simulink model "ThreePhaseASMSaturation"  (R2023b)
settings: Solver=ode23tb  StartTime=0.0  StopTime=3.5  MaxStep=1/60  RelTol=1e-4  AbsTol=1e-4  EnableMultiTasking=on
InitFcn:
  | run('DefaultSimscapeValues.m')
values from neighbouring files (symbols this model uses):
  D = 0    [DefaultSimscapeValues.m]    (also in Newabccoordparam.m = 0.001)
  f = 60    [DefaultSimscapeValues.m]    (also in Newabccoordparam.m = 50)
  J = 1.662    [DefaultSimscapeValues.m]    (also in Newabccoordparam.m = 127)
  Lm = 13.08/377    (= 0.0346949602122)    [DefaultSimscapeValues.m]    (also in Newabccoordparam.m = 0.0025)
  Lr = Lm + Lsi    (= 0.0354960212202)    [DefaultSimscapeValues.m]    (also in Newabccoordparam.m = 0.002587)
  Lri = 0.302/377    (= 0.000801061007958)    [DefaultSimscapeValues.m]    (also in Newabccoordparam.m = 8.7e-05)
  Ls = Lm + Lsi    (= 0.0354960212202)    [DefaultSimscapeValues.m]    (also in Newabccoordparam.m = 0.002587)
  Lsi = 0.302/377    (= 0.000801061007958)    [DefaultSimscapeValues.m]    (also in Newabccoordparam.m = 8.7e-05)
  p = 2    [DefaultSimscapeValues.m]    (also in Newabccoordparam.m)
  Ps = 37300    [DefaultSimscapeValues.m]    (also in Newabccoordparam.m = 2000000)
  Rr = 0.228    [DefaultSimscapeValues.m]    (also in Newabccoordparam.m = 0.0029)
  Rs = 0.087    [DefaultSimscapeValues.m]    (also in Newabccoordparam.m = 0.0026)
  sigma = 1- Lm^2/(Ls*Lr)    (= 0.0446259584738)    [DefaultSimscapeValues.m]    (also in Newabccoordparam.m = 0.0661284179513)
  Vs = 460    [DefaultSimscapeValues.m]    (also in Newabccoordparam.m = 690)
undefined symbols (not defined in the file or in its folder): DiscIntNeverNeededParam
libraries: eeGeneralControl x4, spsabctodq0Lib x4, spsdq0toabcLib x4, spsAsynchronousMachineSIUnitsLib x2, spsThreePhaseProgrammableVoltageSourceLib x1, spsGroundLib x1, sps_lib x1
settings Model: FPTRunName=Active  Creator=The MathWorks, Inc.  LastModifiedBy=collins
settings SolverCC: AutoScaleAbsTol=off  AlgebraicLoopSolver=TrustRegion
settings DataIOCC: LimitDataPoints=on  SaveFormat=Array  ReturnWorkspaceOutputs=off
settings OptimizationCC: ExpressionDepthLimit=2147483647  InitFltsAndDblsToZero=on  EfficientMapNaN2IntZero=off  LifeSpan=inf
settings DebuggingCC: UnderspecifiedInitializationDetection=Classic  MergeDetectMultiDrivingBlocksExec=none  SignalResolutionControl=TryResolveAllWithWarning  SolverPrmCheckMsg=warning  MultiTaskDSMMsg=warning  MultiTaskCondExecSysMsg=none  SigSpecEnsureSampleTimeMsg=none  FcnCallInpInsideContextMsg=warning  UnconnectedInputMsg=warning  UnconnectedOutputMsg=warning  UnconnectedLineMsg=warning  StateNameClashWarn=warning  SFUnexpectedBacktrackingDiag=warning  SFNoUnconditionalDefaultTransitionDiag=warning  SFExecutionAtInitializationDiag=none  ArithmeticOperatorsInVariantConditions=warning
settings HardwareCC: ProdBitPerPointer=32  ProdBitPerSizeT=32  ProdBitPerPtrDiffT=32  ProdLargestAtomicFloat=None  ProdIntDivRoundTo=Undefined  ProdEndianess=Unspecified  ProdWordSize=32  ProdHWDeviceType=32-bit Generic
settings ModelReferenceCC: EnableRefExpFcnMdlSchedulingChecks=on  PropagateSignalLabelsOutOfModel=off
settings SFSimCC: SimUseLocalCustomCode=off  CustomCodeUndefinedFunction=UseInterfaceOnly
settings RTWCC: RTWUseLocalCustomCode=off  DLArmComputeVersion=19.05
settings CodeAppCC: StateflowObjectComments=on
settings GRTTargetCC: TargetLangStandard=C89/C90 (ANSI)  CombineOutputUpdateFcns=off  GRTInterface=on
settings ConfigComp: CovMetricSettings=dw  CovSaveCumulativeToWorkspaceVar=on  CovSaveSingleToWorkspaceVar=on  CovExternalEMLEnable=off  CovSFcnEnable=off
settings SimscapeCC: SimscapeNormalizeSystem=off

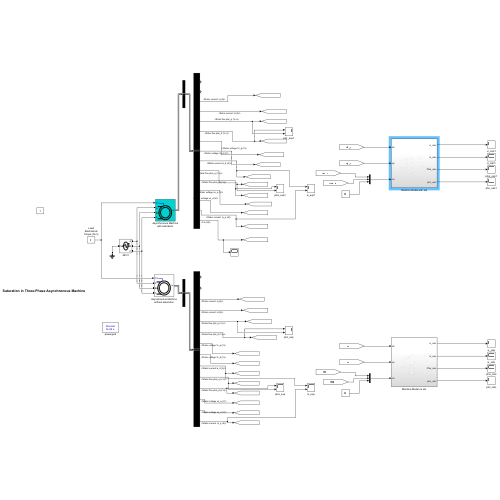
[thumbnail: Simulink's stored preview of the top-level diagram]
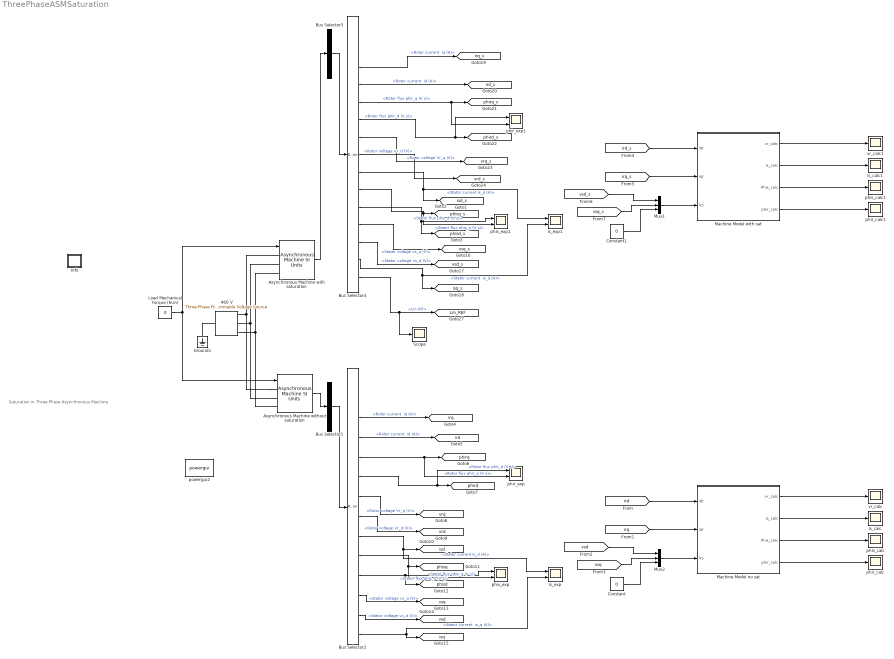
== system ThreePhaseASMSaturation ==
  note: Saturation in Three-Phase Asynchronous Machine
  460 V : spsThreePhaseProgrammableVoltageSourceLib/Three-Phase Programmable Voltage Source  PositiveSequence="[460  0 60]"  VariationEntity=None  VariationType=Step  VariationTypeAlt=Step  VariationStep=0.5  VariationRate=10  VariationMagnitude=0.3  VariationFrequency=2  VariationTiming=[1 2]  VariationPhaseA=off  Amplitudes=[1 0.8 1.2 1.0]  TimeValues=[0 0.1 0.15 0.2]  HarmonicGeneration=off  HarmonicA=[3 0.2 -25 0]  HarmonicB=[2 0.15 35 2]  Timing="[0.05  3]"  BusType=swing  Pref=0  Qref=0  Qmin=-inf  Qmax=inf
  Asynchronous Machine with saturation : spsAsynchronousMachineSIUnitsLib/Asynchronous Machine SI Units  RotorType=Squirrel-cage  PresetModel=No  MechanicalLoad=Torque Tm  ShowDetailedParameters=on  ReferenceFrame=Synchronous  Units=SI  MeasurementBus=off  NominalParameters=[Ps Vs f]  VoltageRatio=1  Stator=[Rs Lsi]  Rotor=[Rr Lri]  Cage1=[ 0.022 0.226/377]  Cage2=[ 0.022 0.226/377]  Lm=13.08/377  Mechanical=[J D p]  PolePairs=2  InitialConditions="[ 1,0   0,0,0   0,0,0 ]"  SimulateSaturation=on  Saturation=[9.9249,19.6672,38.0377,51.3988,69.2824,105.1337,152.5532,214.2421,302;230, 322, 414, 460, 506, 552, 598, 644, 690]  LoadFlowParameters=0  TsPowergui=0  TsBlock=-1  IterativeModel=Trapezoidal non iterative  IterativeDiscreteModel=Trapezoidal non iterative  Pmec=0
  Asynchronous Machine without saturation : spsAsynchronousMachineSIUnitsLib/Asynchronous Machine SI Units  RotorType=Squirrel-cage  PresetModel=No  MechanicalLoad=Torque Tm  ShowDetailedParameters=on  ReferenceFrame=Synchronous  Units=SI  MeasurementBus=off  NominalParameters=[Ps Vs f]  VoltageRatio=1  Stator=[Rs Lsi]  Rotor=[Rr Lri]  Cage1=[ 0.022 0.226/377]  Cage2=[ 0.022 0.226/377]  Lm=Lm  Mechanical=[J D p]  PolePairs=2  InitialConditions=[ 1,0,0,0,0,0,0,0 ]  SimulateSaturation=off  Saturation=[9.9249,19.6672,38.0377,51.3988,69.2824,105.1337,152.5532,214.2421,302;230, 322, 414, 460, 506, 552, 598, 644, 690]  LoadFlowParameters=0  TsPowergui=0  TsBlock=-1  IterativeModel=Trapezoidal non iterative  IterativeDiscreteModel=Trapezoidal non iterative  Pmec=0
  Bus Selector1 : BusSelector  OutputSignals="Stator measurements.Stator current is_a (A),Mechanical.Rotor speed (wm),Rotor measurements.Rotor current  iq (A),Rotor measurements.Rotor current  id (A),Rotor measurements.Rotor flux phir_q (V s),Rotor measurements.Rotor flux phir_d (V s),Rotor measurements.Rotor voltage Vr_q (V),Rotor measurements.Rotor voltage Vr_d (V),Stator measurements.Stator current is_d (A),Stator measurements.Stator flux phis_q (V s),Stator measurements.Stator flux phis_d (V s),Stator measurements.Stator voltage vs_q (V),Stator measurements.Stator voltage vs_d (V),Stator measurements.Stator current  is_q (A)"  OutputAsBus=on
  Bus Selector2 : BusSelector  OutputSignals="Stator current is_a (A),Rotor speed (wm),Rotor current  iq (A),Rotor current  id (A),Rotor flux phir_q (V s),Rotor flux phir_d (V s),Rotor voltage Vr_q (V),Rotor voltage Vr_d (V),Stator current is_d (A),Stator flux phis_q (V s),Stator flux phis_d (V s),Stator voltage vs_q (V),Stator voltage vs_d (V),Stator current  is_q (A)"
  Bus Selector3 : BusSelector  OutputSignals="Stator measurements.Stator current is_a (A),Mechanical.Rotor speed (wm),Rotor measurements.Rotor current  iq (A),Rotor measurements.Rotor current  id (A),Rotor measurements.Rotor flux phir_q (V s),Rotor measurements.Rotor flux phir_d (V s),Rotor measurements.Rotor voltage Vr_q (V),Rotor measurements.Rotor voltage Vr_d (V),Stator measurements.Stator current is_d (A),Stator measurements.Stator flux phis_q (V s),Stator measurements.Stator flux phis_d (V s),Stator measurements.Stator voltage vs_q (V),Stator measurements.Stator voltage vs_d (V),Stator measurements.Stator current  is_q (A),Lm (H)"  OutputAsBus=on
  Bus Selector4 : BusSelector  OutputSignals="Stator current is_a (A),Rotor speed (wm),Rotor current  iq (A),Rotor current  id (A),Rotor flux phir_q (V s),Rotor flux phir_d (V s),Rotor voltage Vr_q (V),Rotor voltage Vr_d (V),Stator current is_d (A),Stator flux phis_q (V s),Stator flux phis_d (V s),Stator voltage vs_q (V),Stator voltage vs_d (V),Stator current  is_q (A),Lm (H)"
  Constant : Constant  Value=0
  Constant1 : Constant  Value=0
  Ground1 : spsGroundLib/Ground  LConnTagsString=a
  Info : Subsystem
      settings: OpenFcn="showExample(\"simscapeelectricalsps/ThreePhaseASMSaturationExample\")"
      mask Display: disp('?')
  Load Mechanical Torque (N.m) : Constant  Value=0
  Machine Model no sat : Subsystem
  Machine Model with sat : Subsystem
  Mux1 : Mux  Inputs=3
  Mux2 : Mux  Inputs=3
  Scope : Scope
  is_calc : Scope
  is_calc1 : Scope
  is_exp : Scope  NumInputPorts=2
  is_exp1 : Scope  NumInputPorts=2
  phir_calc : Scope
  phir_calc1 : Scope
  phir_exp : Scope  NumInputPorts=2
  phir_exp1 : Scope  NumInputPorts=2
  phis_calc : Scope
  phis_calc1 : Scope
  phis_exp : Scope  NumInputPorts=2
  phis_exp1 : Scope  NumInputPorts=2
  powergui2 : sps_lib/powergui  Priority=1  SimulationMode=Discrete  SampleTime=5e-6  frequency=60  Iterations=50  frequencyindice=60  Pbase=100e6  ErrMax=1e-4  UnitsV=kV  UnitsW=MW  buscounter=0  FunctionMessages=off  echomessages=off  EnableUseOfTLC=off  CurrentSourceSwitches=off  DisableSnubberDevices=off  DisableRonSwitches=off  DisableVfSwitches=off  DisplayEquations=off  AutomaticDiscreteSolvers=off  SolverType=Tustin  Interpol=off  ExternalGateDelay=off  methode=off  Ts=0  x0status=blocks  SPID=off  SwTol=0  HookPort=off  NonlinearTolerance=1e-4  nMaxIteration=100  ContinueOnMaxIteration=off  RestoreLinks=warning  ResistiveCurrentMeasurement=off  Frange=[0:2:500]  Ylog=off  Xlog=on  ShowGrid=off  save=off  variable=ZData  structure=0  ZoomFFT=off  StartTime=0.0  cycles=1  DisplayStyle=1  fundamental=60  FreqAxis=off  MaxFrequency=1000  frequencyindicesteady=1  RmsSteady=1  display=off
  vr_calc : Scope
  vr_calc1 : Scope
  tag scope: Lm_REF=global, ird=global, ird_s=global, irq=global, irq_s=global, isd=global, isd_s=global, isq=global, isq_s=global, phird=global, phird_s=global, phirq=global, phirq_s=global, phisd=global, phisd_s=global, phisq=global, phisq_s=global, vrd=global, vrd_s=global, vrq=global, vrq_s=global, vsd=global, vsd_s=global, vsq=global, vsq_s=global
  wires:
  Load Mechanical Torque (N.m)/1 -> Asynchronous Machine with saturation/1, Asynchronous Machine without saturation/1
  Asynchronous Machine without saturation/1 -> Bus Selector1/1
  Machine Model no sat/1(vr_calc) -> vr_calc/1
  Machine Model no sat/2(is_calc) -> is_calc/1
  Machine Model no sat/3(Phis_calc) -> phis_calc/1
  Machine Model no sat/4(phir_calc) -> phir_calc/1
  Bus Selector1/1 -> Bus Selector2/1
  Bus Selector2/3 -> [irq]  "<Rotor current  iq (A)>"
  Bus Selector2/4 -> [ird]  "<Rotor current  id (A)>"
  Bus Selector2/5 -> phir_exp/2, [phirq]  "<Rotor flux phir_q (V s)>"
  Bus Selector2/6 -> phir_exp/1, [phird]  "<Rotor flux phir_d (V s)>"
  Bus Selector2/7 -> [vrq]  "<Rotor voltage Vr_q (V)>"
  Bus Selector2/8 -> [vrd]  "<Rotor voltage Vr_d (V)>"
  Bus Selector2/9 -> is_exp/1, [isd]  "<Stator current is_d (A)>"
  Bus Selector2/10 -> phis_exp/2, [phisq]  "<Stator flux phis_q (V s)>"
  Bus Selector2/11 -> [phisd], phis_exp/1  "<Stator flux phis_d (V s)>"
  Bus Selector2/12 -> [vsq]  "<Stator voltage vs_q (V)>"
  Bus Selector2/13 -> [vsd]  "<Stator voltage vs_d (V)>"
  Bus Selector2/14 -> [isq], is_exp/2  "<Stator current  is_q (A)>"
  Constant/1 -> Mux2/3
  Mux2/1 -> Machine Model no sat/3(Vs)
  [ird] -> Machine Model no sat/1(idr)
  [irq] -> Machine Model no sat/2(iqr)
  [vsd] -> Mux2/1
  [vsq] -> Mux2/2
  [vsq_s] -> Mux1/2
  [irq_s] -> Machine Model with sat/2(iqr)
  Bus Selector4/4 -> [ird_s]  "<Rotor current  id (A)>"
  Bus Selector4/7 -> [vrq_s]  "<Rotor voltage Vr_q (V)>"
  Mux1/1 -> Machine Model with sat/3(Vs)
  Constant1/1 -> Mux1/3
  Bus Selector3/1 -> Bus Selector4/1
  Bus Selector4/3 -> [irq_s]  "<Rotor current  iq (A)>"
  Bus Selector4/8 -> [vrd_s]  "<Rotor voltage Vr_d (V)>"
  Bus Selector4/14 -> [isq_s], is_exp1/2  "<Stator current  is_q (A)>"
  Bus Selector4/9 -> [isd_s], is_exp1/1  "<Stator current is_d (A)>"
  Bus Selector4/13 -> [vsd_s]  "<Stator voltage vs_d (V)>"
  Bus Selector4/6 -> phir_exp1/1, [phird_s]  "<Rotor flux phir_d (V s)>"
  Bus Selector4/10 -> phis_exp1/2, [phisq_s]  "<Stator flux phis_q (V s)>"
  Machine Model with sat/1(vr_calc) -> vr_calc1/1
  Bus Selector4/12 -> [vsq_s]  "<Stator voltage vs_q (V)>"
  Bus Selector4/5 -> phir_exp1/2, [phirq_s]  "<Rotor flux phir_q (V s)>"
  Machine Model with sat/3(Phis_calc) -> phis_calc1/1
  Machine Model with sat/4(phir_calc) -> phir_calc1/1
  [vsd_s] -> Mux1/1
  Machine Model with sat/2(is_calc) -> is_calc1/1
  Asynchronous Machine with saturation/1 -> Bus Selector3/1
  Bus Selector4/11 -> [phisd_s], phis_exp1/1  "<Stator flux phis_d (V s)>"
  [ird_s] -> Machine Model with sat/1(idr)
  Bus Selector4/15 -> Scope/1, [Lm_REF]  "<Lm (H)>"
  connections:
  Asynchronous Machine without saturation/LConn1 -- Asynchronous Machine with saturation/LConn1 -- 460 V/RConn1
  460 V/RConn2 -- Asynchronous Machine without saturation/LConn2 -- Asynchronous Machine with saturation/LConn2
  460 V/RConn3 -- Asynchronous Machine without saturation/LConn3 -- Asynchronous Machine with saturation/LConn3
  Ground1/LConn1 -- 460 V/LConn1

== system ThreePhaseASMSaturation/Info ==

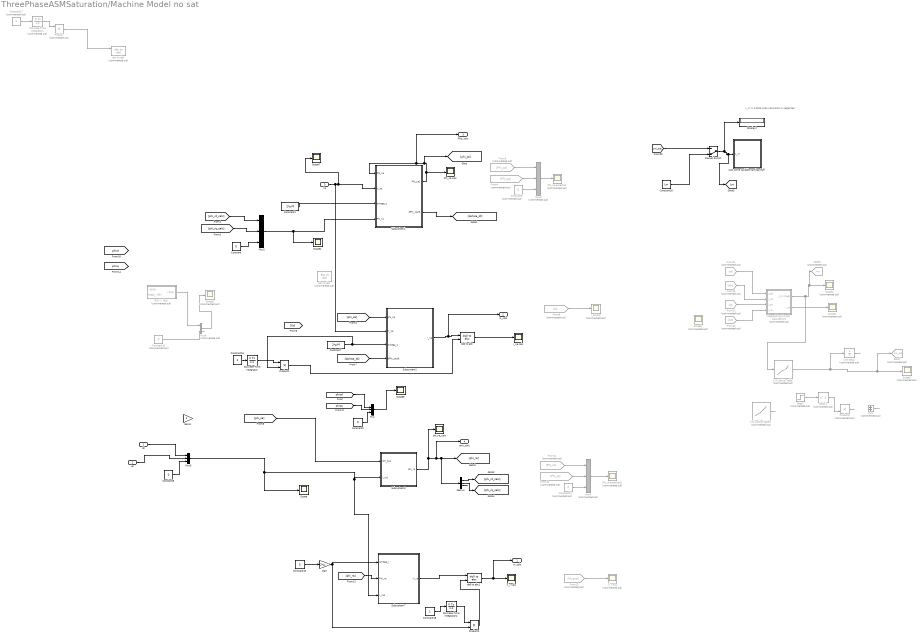
== system ThreePhaseASMSaturation/Machine Model no sat ==
  note: L_m = 0.0025 when saturation is neglected
  idr : Inport
  iqr : Inport  Port=2
  Vs : Inport  Port=3
  1-D Lookup Table : Lookup_n-D  Commented=on  NumberOfTableDimensions=1  BreakpointsForDimension1=[11.2 14.33 18.33 21.31 24.42 26.74 29.07 33.21 40.78 46.21 53.21 60.33 66.1 10000]  Table=|  InternalRulePriority=Speed  RndMeth=Simplest
      | [0.033928571
      | 0.033928571
      | 0.031948882
      | 0.03
      | 0.026845638
      | 0.022508039
      | 0.017241379
      | 0.012875536
      | 0.009661836
      | 0.007926024
      | 0.007366483
      | 0.007142857
      | 0.007022472
      | 0.007]
  1-D Lookup Table1 : Lookup_n-D  Commented=on  NumberOfTableDimensions=1  BreakpointsForDimension1=[11.2 14.33 18.33 21.31 24.42 26.74 29.07 33.21 40.78 46.21 53.21 60.33 66.1 10000]  Table=|  InternalRulePriority=Speed  RndMeth=Simplest
      | [0.033928571
      | 0.033928571
      | 0.031948882
      | 0.03
      | 0.026845638
      | 0.022508039
      | 0.017241379
      | 0.012875536
      | 0.009661836
      | 0.007926024
      | 0.007366483
      | 0.007142857
      | 0.007022472
      | 0.007]
  Constant : Constant  Value=0
  Constant1 : Constant  Value=2*pi*f
  Constant10 : Constant  Commented=on  Value=0
  Constant11 : Constant  Commented=on  Value=0
  Constant15 : Constant  Value=5
  Constant16 : Constant
  Constant17 : Constant  Commented=on
  Constant18 : Constant
  Constant2 : Constant  Value=0
  Constant20 : Constant  Value=Lm
  Constant6 : Constant  Commented=on  Value=0
  Constant7 : Constant  Value=2*pi*f
  Constant8 : Constant  Value=0
  "D/Q -> d/q1" : Subsystem  Commented=on
  Delay1 : Delay  Commented=on  DelayLength=1  SampleTime=15e-5
  Demux : Demux  Outputs=3
  Discrete-Time Integrator : DiscreteIntegrator  SampleTime=-1  ICPrevOutput=DiscIntNeverNeededParam  ICPrevScaledInput=DiscIntNeverNeededParam
  Discrete-Time Integrator1 : DiscreteIntegrator  Commented=on  SampleTime=-1  ICPrevOutput=DiscIntNeverNeededParam  ICPrevScaledInput=DiscIntNeverNeededParam
  Discrete-Time Integrator2 : DiscreteIntegrator  SampleTime=-1  ICPrevOutput=DiscIntNeverNeededParam  ICPrevScaledInput=DiscIntNeverNeededParam
  Display2 : Display
  From10 : From  Commented=on  GotoTag=Phi_rq
  From11 : From  Commented=on  GotoTag=Phi_rd
  From13 : From  Commented=on  GotoTag=Vr_exp
  From15 : From  Commented=on  GotoTag=idr  TagVisibility=global
  From20 : From  Commented=on  GotoTag=iqr  TagVisibility=global
  From21 : From  Commented=on  GotoTag=isd
  From22 : From  Commented=on  GotoTag=isq
  From4 : From  Commented=on  GotoTag=Phi_sq
  From5 : From  Commented=on  GotoTag=Phi_sd
  From9 : From  Commented=on  GotoTag=Is
  Gain : Gain  Gain=2*pi
  Gain3 : Gain
  Goto6 : Goto  Commented=on  GotoTag=Im  TagVisibility=global
  Goto7 : Goto  Commented=on  GotoTag=Lm_sat  TagVisibility=global
  Just some variable naming stuff : Subsystem
  Magnetising Current Calculations : Subsystem  Commented=on
  Manual Switch : ManualSwitch  CurrentSetting=0
  Mux : Mux  Inputs=3
  Mux2 : Mux  Inputs=3
  Mux3 : Mux  Commented=on  Inputs=3
  Mux4 : Mux  Commented=on  Inputs=3
  Mux5 : Mux  Inputs=3
  Mux6 : Mux  Commented=on  Inputs=2
  Phi_ra expected1 : Scope  Commented=on
  Phi_sa calc : Scope
  Phi_sa expected : Scope  Commented=on
  Product : Product  Commented=on
  Product1 : Product
  Product2 : Product
  Product5 : Product  Commented=on
  Scope{,1,7..8} (4 alike) : Scope
  Scope{2..6} (5 alike) : Scope  Commented=on
  Step3 : Step  Commented=on  Time=0  SampleTime=0
  Subsystem1 : Subsystem
  Subsystem2 : Subsystem
  Subsystem3 : Subsystem
  Subsystem7 : Subsystem
  Sum : Sum  Commented=on  Inputs=|++
  Unit Delay : UnitDelay  Commented=on  InitialCondition=0.034  SampleTime=-1  HasFrameUpgradeWarning=on
  V_r calc : Scope
  V_r exp : Scope  Commented=on
  abc to dq0 : spsabctodq0Lib/abc to dq0  Commented=on  Alignment=90 degrees behind phase A axis
  abc to dq2 : spsabctodq0Lib/abc to dq0  Commented=on  Alignment=90 degrees behind phase A axis
  dq0 to abc : spsdq0toabcLib/dq0 to abc  Alignment=90 degrees behind phase A axis
  dq0 to abc1 : spsdq0toabcLib/dq0 to abc  Alignment=Aligned with phase A axis
  i_sa calc : Scope
  i_sa exp : Scope  Commented=on
  phi_ra_calc : Scope
  vr_calc : Outport
  is_calc : Outport  Port=2
  Phis_calc : Outport  Port=3
  phir_calc : Outport  Port=4
  tag scope: Lm=global
  wires:
  Magnetising Current Calculations/1(i_m (mag)) -> 1-D Lookup Table/1, Goto6/1, Scope4/1
  ? -> Sum/2
  Manual Switch/1 -> [Lm], Just some variable naming stuff/1(L_m), Display2/1
  Constant6/1 -> Mux3/3
  Demux/1 -> [phi_rd_calc]
  Constant11/1 -> Mux4/3
  Discrete-Time Integrator2/1 -> Product2/1
  Product1/1 -> dq0 to abc/2
  Constant18/1 -> Discrete-Time Integrator2/1
  Mux5/1 -> Subsystem7/3(i_ra1), Subsystem3/2(i_ra1), Scope/1
  Discrete-Time Integrator/1 -> Product1/1
  From5/1 -> Mux3/1
  Sum/1 -> ?
  "D/Q -> d/q1"/1(i dr/qr) -> Mux6/1
  Subsystem3/1(phi_ra) -> phir_calc/1, Demux/1, [phi_ra], phi_ra_calc/1
  dq0 to abc/1 -> i_sa calc/1
  [phi_sa] -> Subsystem2/1(phi_sa)
  Delay1/1 -> Product5/2
  Constant8/1 -> Mux5/3
  Discrete-Time Integrator1/1 -> Product/1
  Subsystem2/1(i_sa) -> is_calc/1, dq0 to abc/1
  From15/1 -> Magnetising Current Calculations/2(i_rd)
  Demux/2 -> [phi_rq_calc]
  Constant1/1 -> Subsystem1/3(omega_s)
  1-D Lookup Table/1 -> Unit Delay/1, Goto7/1, Scope5/1
  Constant20/1 -> Manual Switch/2
  From22/1 -> Magnetising Current Calculations/3(i_sq)
  From9/1 -> i_sa exp/1
  From21/1 -> Magnetising Current Calculations/1(i_sd)
  Subsystem1/1(Phi_sa1) -> Phi_sa calc/1, [phi_sa], Phis_calc/1, Subsystem1/1(Phi_sa)
  From11/1 -> Mux4/1
  From20/1 -> Magnetising Current Calculations/4(i_rq)
  Subsystem7/1(V_ra) -> dq0 to abc1/1
  Mux6/1 -> Scope3/1
  [Lm_sat] -> Manual Switch/1
  ? -> Scope6/1
  Subsystem1/2(dPhi_sa/dt) -> [dphisa_dt]
  From13/1 -> V_r exp/1
  [phi_ra] -> Subsystem7/2(Phi_ra)
  Product/1 -> abc to dq0/1
  Constant17/1 -> Discrete-Time Integrator1/1
  Step3/1 -> Delay1/1
  Product2/1 -> dq0 to abc1/2
  [dphisa_dt] -> Subsystem2/4(dPhi_sa/dt)
  From10/1 -> Mux4/2
  Mux3/1 -> Phi_sa expected/1
  From4/1 -> Mux3/2
  Constant/1 -> Mux2/3
  ? -> 1-D Lookup Table1/1
  Magnetising Current Calculations/2(i_m) -> Scope2/1
  Constant15/1 -> Gain/1
  dq0 to abc1/1 -> vr_calc/1, V_r calc/1
  Mux2/1 -> Scope1/1, Subsystem1/4(Phi_ra)
  Gain/1 -> Subsystem7/1(omega_r), Product2/2
  Constant16/1 -> Discrete-Time Integrator/1
  Constant10/1 -> ?
  ? -> Mux6/2
  Mux4/1 -> Phi_ra expected1/1
  ? -> Product5/1
  Product5/1 -> ?
  Demux/3 -> ?
  ? -> Sum/1
  1-D Lookup Table1/1 -> ?
  Unit Delay/1 -> ?
  ? -> "D/Q -> d/q1"/2(theta_r (θr))
  Vs/1 -> Subsystem1/2(V_sa), Scope7/1, Subsystem2/2(V_sa)
  Constant2/1 -> Mux/3
  Mux/1 -> Scope8/1
  [phisd] -> Mux/1
  [phisq] -> Mux/2
  idr/1 -> Mux5/1
  iqr/1 -> Mux5/2
  [phi_rd_calc] -> Mux2/1
  [phi_rq_calc] -> Mux2/2
  Constant7/1 -> Product1/2, Subsystem2/3(omega_s)
  [phi_sa] -> Subsystem3/1(phi_sa1)

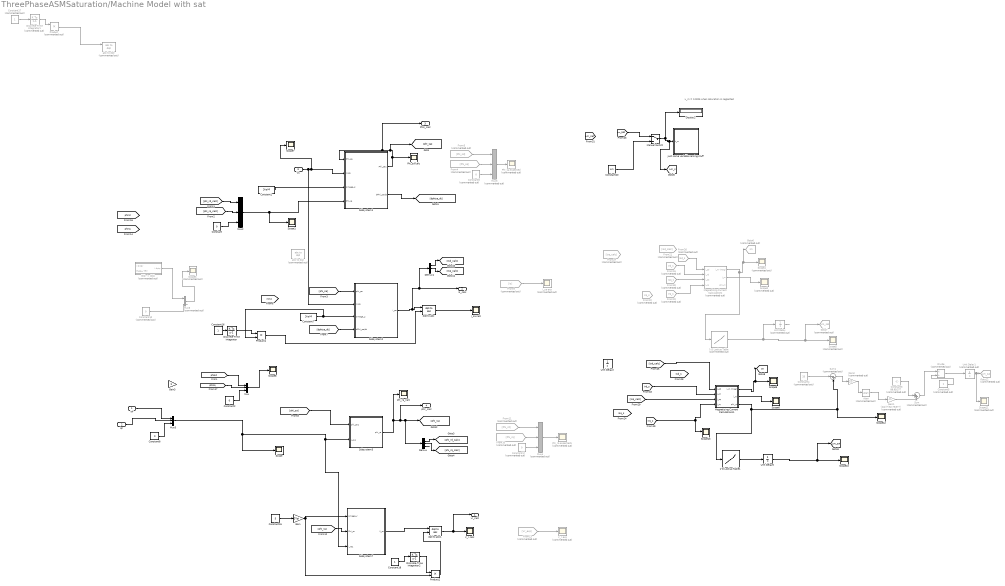
== system ThreePhaseASMSaturation/Machine Model with sat ==
  note: L_m = 0.0025 when saturation is neglected
  idr : Inport
  iqr : Inport  Port=2
  Vs : Inport  Port=3
  1-D Lookup Table : Lookup_n-D  Commented=on  NumberOfTableDimensions=1  BreakpointsForDimension1=|  Table=|  InternalRulePriority=Speed  RndMeth=Simplest
      BreakpointsForDimension1=|
      | [0
      | 14.03592819
      | 27.81362097
      | 53.79343122
      | 72.68888005
      | 97.98010971
      | 148.6815044
      | 215.7428044
      | 302.9840835
      | 427.0924958
      | ]
      Table=|
      | [0.03469496
      | 0.025049278
      | 0.01328421
      | 0.009132391
      | 0.006822943
      | 0.003403469
      | 0.002573177
      | 0.00197797
      | 0.001390402
      | 0.001390402
      | ]
  1-D Lookup Table1 : Lookup_n-D  NumberOfTableDimensions=1  BreakpointsForDimension1=|  Table=|  InternalRulePriority=Speed  RndMeth=Simplest
      BreakpointsForDimension1=|
      | [0
      | 0.05
      | 0.1
      | 0.15
      | 0.2
      | 0.25
      | 0.3
      | 0.35
      | 0.4
      | 0.45
      | 0.5
      | 0.55
      | 0.6
      | 0.65
      | 0.7
      | 0.75
      | 0.8
      | 0.85
      | 0.9
      | 0.95
      | 1
      | 1.05
      | 1.1
      | 1.15
      | 1.2
      | 1.25
      | 1.3
      | 1.35
      | 1.4
      | 1.45
      | 1.5
      | 1.55
      | 1.6
      | 1.65
      | 1.7
      | 1.75
      | 1.8
      | 1.85
      | 1.9
      | 1.95
      | 2
      | 2.05
      | 2.1
      | 2.15
      | 2.2
      | 2.25
      | 2.3
      | ]
      Table=|
      | [0.034924939
      | 0.034733822
      | 0.03451881
      | 0.034275134
      | 0.033996668
      | 0.033675415
      | 0.033300731
      | 0.032858148
      | 0.032327492
      | 0.031679798
      | 0.030872018
      | 0.029837483
      | 0.02846779
      | 0.026576553
      | 0.023825934
      | 0.019616436
      | 0.013559401
      | 0.009046612
      | 0.007728863
      | 0.007297556
      | 0.007098429
      | 0.006985741
      | 0.006913676
      | 0.006863749
      | 0.006827163
      | 0.006799221
      | 0.006777193
      | 0.006759385
      | 0.006744693
      | 0.006732367
      | 0.006721879
      | 0.006712846
      | 0.006704986
      | 0.006698085
      | 0.006691977
      | 0.006686533
      | 0.006681651
      | 0.006677248
      | 0.006673256
      | 0.006669621
      | 0.006666298
      | 0.006663246
      | 0.006660436
      | 0.006657838
      | 0.00665543
      | 0.006653192
      | 0.006651107]
  Atan : Trigonometry  Commented=on  Operator=atan
  Constant : Constant  Value=0
  Constant1 : Constant  Value=2*pi*f
  Constant10 : Constant  Commented=on  Value=0
  Constant11 : Constant  Commented=on  Value=0
  Constant15 : Constant  Value=5
  Constant16 : Constant
  Constant17 : Constant  Commented=on
  Constant18 : Constant
  Constant2 : Constant  Value=0
  Constant20 : Constant  Value=Lm
  Constant3 : Constant  Commented=on  Value=88.95/377
  Constant4 : Constant  Commented=on  Value=20
  Constant5 : Constant  Commented=on
  Constant6 : Constant  Commented=on  Value=0
  Constant7 : Constant  Value=2*pi*f
  Constant8 : Constant  Value=0
  "D/Q -> d/q1" : Subsystem  Commented=on
  Demux : Demux  Outputs=3
  Demux1 : Demux  Outputs=3
  Discrete-Time Integrator : DiscreteIntegrator  SampleTime=-1  ICPrevOutput=DiscIntNeverNeededParam  ICPrevScaledInput=DiscIntNeverNeededParam
  Discrete-Time Integrator1 : DiscreteIntegrator  Commented=on  SampleTime=-1  ICPrevOutput=DiscIntNeverNeededParam  ICPrevScaledInput=DiscIntNeverNeededParam
  Discrete-Time Integrator2 : DiscreteIntegrator  SampleTime=-1  ICPrevOutput=DiscIntNeverNeededParam  ICPrevScaledInput=DiscIntNeverNeededParam
  Display2 : Display
  Divide : Product  Commented=on  Inputs=*/
  From10 : From  Commented=on  GotoTag=Phi_rq
  From11 : From  Commented=on  GotoTag=Phi_rd
  From13 : From  Commented=on  GotoTag=Vr_exp
  From15 : From  Commented=on  GotoTag=ird_s  TagVisibility=global
  From20 : From  Commented=on  GotoTag=irq_s  TagVisibility=global
  From21 : From  Commented=on  GotoTag=isd_calc
  From22 : From  Commented=on  GotoTag=irq_s  TagVisibility=global
  From26 : From  Commented=on  GotoTag=isd_s  TagVisibility=global
  From27 : From  Commented=on  GotoTag=isq_calc
  From30 : From  Commented=on  GotoTag=isq_s  TagVisibility=global
  From4 : From  Commented=on  GotoTag=Phi_sq
  From5 : From  Commented=on  GotoTag=Phi_sd
  From9 : From  Commented=on  GotoTag=Is
  Gain : Gain  Gain=2*pi
  Gain1 : Gain  Commented=on  Gain=(2/pi)*(62.75/377)
  Gain2 : Gain  Commented=on  Gain=20
  Gain3 : Gain
  Goto12 : Goto  Commented=on  GotoTag=Lm_sat  TagVisibility=global
  Goto6 : Goto  Commented=on  GotoTag=Im  TagVisibility=global
  Goto7 : Goto  Commented=on  GotoTag=Lm_sat  TagVisibility=global
  Just some variable naming stuff : Subsystem
  Magnetising Current Calculations : Subsystem  Commented=on
  Magnetising Current Calculations1 : Subsystem
  Manual Switch : ManualSwitch
  Mux : Mux  Inputs=3
  Mux2 : Mux  Inputs=3
  Mux3 : Mux  Commented=on  Inputs=3
  Mux4 : Mux  Commented=on  Inputs=3
  Mux5 : Mux  Inputs=3
  Mux6 : Mux  Commented=on  Inputs=2
  Phi_ra expected1 : Scope  Commented=on
  Phi_sa calc : Scope
  Phi_sa expected : Scope  Commented=on
  Product : Product  Commented=on
  Product1 : Product
  Product2 : Product
  Scope{,1,6..10,12} (8 alike) : Scope
  Scope{2..5,11} (5 alike) : Scope  Commented=on
  Scope13 : Scope  NumInputPorts=2
  Subsystem1 : Subsystem
  Subsystem2 : Subsystem
  Subsystem3 : Subsystem
  Subsystem7 : Subsystem
  Sum : Sum  Commented=on  Inputs=|++
  Sum1 : Sum  Commented=on  Inputs=|-+
  Unit Delay : UnitDelay  Commented=on  InitialCondition=0.034  SampleTime=-1  HasFrameUpgradeWarning=on
  Unit Delay1 : UnitDelay  Commented=on  InitialCondition=0.034  SampleTime=-1  HasFrameUpgradeWarning=on
  Unit Delay2 : UnitDelay  SampleTime=-1  HasFrameUpgradeWarning=on
  Unit Delay6 : UnitDelay  InitialCondition=0.034  SampleTime=-1  HasFrameUpgradeWarning=on
  V_r calc : Scope
  V_r exp : Scope  Commented=on
  abc to dq0 : spsabctodq0Lib/abc to dq0  Commented=on  Alignment=90 degrees behind phase A axis
  abc to dq2 : spsabctodq0Lib/abc to dq0  Commented=on  Alignment=90 degrees behind phase A axis
  dq0 to abc : spsdq0toabcLib/dq0 to abc  Alignment=90 degrees behind phase A axis
  dq0 to abc1 : spsdq0toabcLib/dq0 to abc  Alignment=Aligned with phase A axis
  i_sa calc : Scope
  i_sa exp : Scope  Commented=on
  phi_ra_calc : Scope
  vr_calc : Outport
  is_calc : Outport  Port=2
  Phis_calc : Outport  Port=3
  phir_calc : Outport  Port=4
  tag scope: Im=global, Lm_s=global, Lm_sat=global
  wires:
  Manual Switch/1 -> [Lm_s], Just some variable naming stuff/1(L_m), Display2/1
  Constant6/1 -> Mux3/3
  Demux/1 -> [phi_rd_calc]
  Constant11/1 -> Mux4/3
  Discrete-Time Integrator2/1 -> Product2/1
  Product1/1 -> dq0 to abc/2
  Constant18/1 -> Discrete-Time Integrator2/1
  Mux5/1 -> Subsystem7/3(i_ra1), Subsystem3/2(i_ra1), Scope/1
  Discrete-Time Integrator/1 -> Product1/1
  From5/1 -> Mux3/1
  "D/Q -> d/q1"/1(i dr/qr) -> Mux6/1
  Subsystem3/1(phi_ra) -> phir_calc/1, Demux/1, [phi_ra], phi_ra_calc/1
  dq0 to abc/1 -> i_sa calc/1
  [phi_sa] -> Subsystem2/1(phi_sa)
  Constant8/1 -> Mux5/3
  Discrete-Time Integrator1/1 -> Product/1
  Subsystem2/1(i_sa) -> Demux1/1, is_calc/1, dq0 to abc/1
  Demux/2 -> [phi_rq_calc]
  Constant1/1 -> Subsystem1/3(omega_s)
  1-D Lookup Table/1 -> Unit Delay/1, Goto7/1, Scope5/1
  Constant20/1 -> Manual Switch/2
  From9/1 -> i_sa exp/1
  Subsystem1/1(Phi_sa1) -> Phi_sa calc/1, [phi_sa], Phis_calc/1, Subsystem1/1(Phi_sa)
  From11/1 -> Mux4/1
  From20/1 -> Magnetising Current Calculations/4(i_rq)
  Subsystem7/1(V_ra) -> dq0 to abc1/1
  Mux6/1 -> Scope3/1
  Subsystem1/2(dPhi_sa/dt) -> [dphisa_dt]
  From13/1 -> V_r exp/1
  [phi_ra] -> Subsystem7/2(Phi_ra)
  Product/1 -> abc to dq0/1
  Constant17/1 -> Discrete-Time Integrator1/1
  Product2/1 -> dq0 to abc1/2
  [dphisa_dt] -> Subsystem2/4(dPhi_sa/dt)
  From10/1 -> Mux4/2
  Mux3/1 -> Phi_sa expected/1
  From4/1 -> Mux3/2
  Constant/1 -> Mux2/3
  Magnetising Current Calculations/2(i_m) -> Scope2/1
  Constant15/1 -> Gain/1
  dq0 to abc1/1 -> vr_calc/1, V_r calc/1
  Mux2/1 -> Scope1/1, Subsystem1/4(Phi_ra)
  Gain/1 -> Subsystem7/1(omega_r), Product2/2
  Constant16/1 -> Discrete-Time Integrator/1
  Constant10/1 -> ?
  ? -> Mux6/2
  Mux4/1 -> Phi_ra expected1/1
  Demux/3 -> ?
  Unit Delay/1 -> ?
  ? -> "D/Q -> d/q1"/2(theta_r (θr))
  Vs/1 -> Subsystem1/2(V_sa), Scope7/1, Subsystem2/2(V_sa)
  Constant2/1 -> Mux/3
  Mux/1 -> Scope8/1
  [phisd] -> Mux/1
  [phisq] -> Mux/2
  idr/1 -> Mux5/1
  iqr/1 -> Mux5/2
  Constant7/1 -> Product1/2, Subsystem2/3(omega_s)
  Magnetising Current Calculations/1(i_m (mag)) -> 1-D Lookup Table/1, Goto6/1, Scope4/1
  Magnetising Current Calculations1/2(i_m) -> Scope6/1
  Magnetising Current Calculations1/1(i_m (mag)) -> [Im], Scope9/1
  Demux1/1 -> [isd_calc]
  Demux1/2 -> [isq_calc]
  From15/1 -> Magnetising Current Calculations/2(i_rd)
  From26/1 -> Magnetising Current Calculations/1(i_sd)
  From30/1 -> Magnetising Current Calculations/3(i_sq)
  Atan/1 -> Gain1/1
  Constant3/1 -> Sum/1
  Sum/1 -> Divide/1
  Sum1/1 -> Gain2/1
  Gain2/1 -> Atan/1
  Gain1/1 -> Sum/2
  Magnetising Current Calculations1/3(phi_m) -> Sum1/2, Scope12/1, 1-D Lookup Table1/1
  Constant4/1 -> Sum1/1
  Unit Delay1/1 -> Scope11/1, Goto12/1
  Constant5/1 -> Divide/2
  Divide/1 -> Unit Delay1/1
  [phi_rd_calc] -> Mux2/1
  [phi_rq_calc] -> Mux2/2
  1-D Lookup Table1/1 -> Unit Delay6/1
  [isq_calc] -> Magnetising Current Calculations1/3(i_sq)
  [isd_calc] -> Magnetising Current Calculations1/1(i_sd)
  Unit Delay6/1 -> [Lm_sat], Scope10/1
  [ird_s] -> Magnetising Current Calculations1/2(i_rd)
  [irq_s] -> Magnetising Current Calculations1/4(i_rq), Scope13/1
  [Lm_REF] -> Manual Switch/1
  [phi_sa] -> Subsystem3/1(phi_sa1)

== system ThreePhaseASMSaturation/Machine Model no sat/D//Q -> d//q1 ==
  i Dr/Qr : Inport
  theta_r (θr) : Inport  Port=2
  Fcn : Fcn  Expr=u[1]*cos(u[3])+u[2]*sin(u[3])
  Fcn1 : Fcn  Expr=-u[1]*sin(u[3])+u[2]*cos(u[3])
  Mux : Mux  Inputs=2
  Mux1 : Mux  Inputs=2
  i dr/qr : Outport  VectorParamsAs1DForOutWhenUnconnected=off
  wires:
  Mux/1 -> i dr/qr/1
  Fcn/1 -> Mux/1
  Fcn1/1 -> Mux/2
  i Dr/Qr/1 -> Mux1/1
  Mux1/1 -> Fcn1/1, Fcn/1
  theta_r (θr)/1 -> Mux1/2

== system ThreePhaseASMSaturation/Machine Model no sat/Just some variable naming stuff ==
  L_m : Inport
  Constant14 : Constant  Value=Lsi
  Constant19 : Constant  Value=Lri
  Constant20 : Constant
  Divide : Product  Inputs=**/
  Product : Product
  Sum : Sum  Inputs=|++
  Sum1 : Sum  Inputs=|++
  Sum2 : Sum  Inputs=|+-
  tag scope: Lr=global, Ls=global, sigma=global
  wires:
  L_m/1 -> Divide/2, Divide/1, Sum/2, Sum1/1
  Constant20/1 -> Sum2/1
  Constant14/1 -> Sum1/2
  Sum/1 -> Product/1, [Lr]
  Divide/1 -> Sum2/2
  Sum2/1 -> [sigma]
  Constant19/1 -> Sum/1
  Sum1/1 -> Product/2, [Ls]
  Product/1 -> Divide/3

== system ThreePhaseASMSaturation/Machine Model no sat/Magnetising Current Calculations ==
  i_sd : Inport
  i_rd : Inport  Port=2
  i_sq : Inport  Port=3
  i_rq : Inport  Port=4
  Mux6 : Mux  Inputs=2
  Sqrt : Sqrt
  Square : Math  Operator=square
  Square1 : Math  Operator=square
  Sum : Sum  Inputs=|++
  Sum1 : Sum  Inputs=|++
  Sum2 : Sum  Inputs=|++
  i_m (mag) : Outport
  i_m : Outport  Port=2
  wires:
  Sum/1 -> Square/1
  Square1/1 -> Mux6/2, Sum2/2
  Sum2/1 -> Sqrt/1
  i_sq/1 -> Sum1/1
  i_rd/1 -> Sum/2
  Square/1 -> Mux6/1, Sum2/1
  Sum1/1 -> Square1/1
  i_sd/1 -> Sum/1
  Mux6/1 -> i_m/1
  Sqrt/1 -> i_m (mag)/1
  i_rq/1 -> Sum1/2

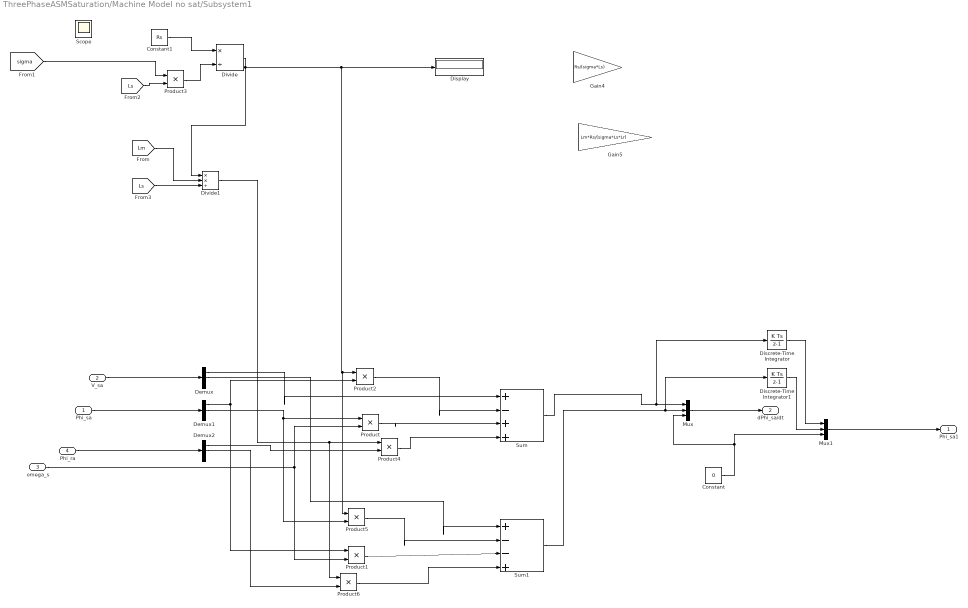
== system ThreePhaseASMSaturation/Machine Model no sat/Subsystem1 ==
  Phi_sa : Inport
  V_sa : Inport  Port=2
  omega_s : Inport  Port=3
  Phi_ra : Inport  Port=4
  Constant : Constant  Value=0
  Constant1 : Constant  Value=Rs
  Demux : Demux  Outputs=3
  Demux1 : Demux  Outputs=3
  Demux2 : Demux  Outputs=3
  Discrete-Time Integrator : DiscreteIntegrator  SampleTime=-1  ICPrevOutput=DiscIntNeverNeededParam  ICPrevScaledInput=DiscIntNeverNeededParam
  Discrete-Time Integrator1 : DiscreteIntegrator  SampleTime=-1  ICPrevOutput=DiscIntNeverNeededParam  ICPrevScaledInput=DiscIntNeverNeededParam
  Display : Display
  Divide : Product  Inputs=*/  OutDataTypeStr=double
  Divide1 : Product  Inputs=**/  OutDataTypeStr=double
  Gain4 : Gain  Gain=Rs/(sigma*Ls)
  Gain5 : Gain  Gain=Lm*Rs/(sigma*Ls*Lr)
  Mux : Mux  Inputs=3
  Mux1 : Mux  Inputs=3
  Product{,1..6} (7 alike) : Product
  Scope : Scope
  Sum : Sum  Inputs=|+-++
  Sum1 : Sum  Inputs=|+--+
  Phi_sa1 : Outport
  dPhi_sa/dt : Outport  Port=2
  wires:
  Product2/1 -> Sum/2
  Product4/1 -> Sum/4
  Product/1 -> Sum/3
  Mux/1 -> dPhi_sa/dt/1
  Demux/1 -> Sum/1
  Product5/1 -> Sum1/2
  Product6/1 -> Sum1/4
  Product1/1 -> Sum1/3
  Demux/2 -> Sum1/1
  Mux1/1 -> Phi_sa1/1
  Demux1/1 -> Product2/2, Product1/1
  Demux2/1 -> Product4/2
  Demux1/2 -> Product5/2, Product/1
  Demux2/2 -> Product6/2
  Constant/1 -> Mux1/3, Mux/3
  Phi_sa/1 -> Demux1/1
  Phi_ra/1 -> Demux2/1
  omega_s/1 -> Product/2, Product1/2
  Sum/1 -> Discrete-Time Integrator/1, Mux/1
  Sum1/1 -> Discrete-Time Integrator1/1, Mux/2
  V_sa/1 -> Demux/1
  [sigma] -> Product3/1
  [Lm] -> Divide1/2
  Divide/1 -> Display/1, Product5/1, Product2/1, Divide1/1
  Constant1/1 -> Divide/1
  [Ls] -> Product3/2
  Product3/1 -> Divide/2
  [Ls] -> Divide1/3
  Divide1/1 -> Product6/1, Product4/1
  Discrete-Time Integrator/1 -> Mux1/1
  Discrete-Time Integrator1/1 -> Mux1/2

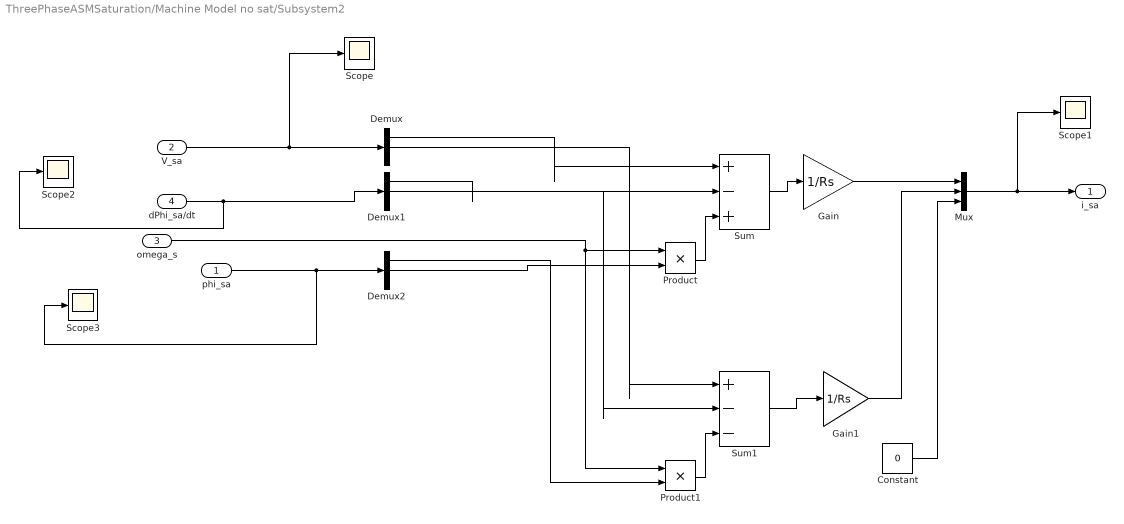
== system ThreePhaseASMSaturation/Machine Model no sat/Subsystem2 ==
  phi_sa : Inport
  V_sa : Inport  Port=2
  omega_s : Inport  Port=3
  dPhi_sa/dt : Inport  Port=4
  Constant : Constant  Value=0
  Demux : Demux  Outputs=3
  Demux1 : Demux  Outputs=3
  Demux2 : Demux  Outputs=3
  Gain : Gain  Gain=1/Rs
  Gain1 : Gain  Gain=1/Rs
  Mux : Mux  Inputs=3
  Product : Product
  Product1 : Product
  Scope{,1..3} (4 alike) : Scope
  Sum : Sum  Inputs=|+-+
  Sum1 : Sum  Inputs=|+--
  i_sa : Outport
  wires:
  Product/1 -> Sum/3
  Constant/1 -> Mux/3
  Demux/1 -> Sum/1
  Demux1/1 -> Sum/2
  Demux2/2 -> Product/2
  Product1/1 -> Sum1/3
  Sum/1 -> Gain/1
  Sum1/1 -> Gain1/1
  Demux/2 -> Sum1/1
  Demux1/2 -> Sum1/2
  Demux2/1 -> Product1/2
  Gain/1 -> Mux/1
  Gain1/1 -> Mux/2
  Mux/1 -> Scope1/1, i_sa/1
  dPhi_sa/dt/1 -> Scope2/1, Demux1/1
  phi_sa/1 -> Scope3/1, Demux2/1
  omega_s/1 -> Product1/1, Product/1
  V_sa/1 -> Scope/1, Demux/1

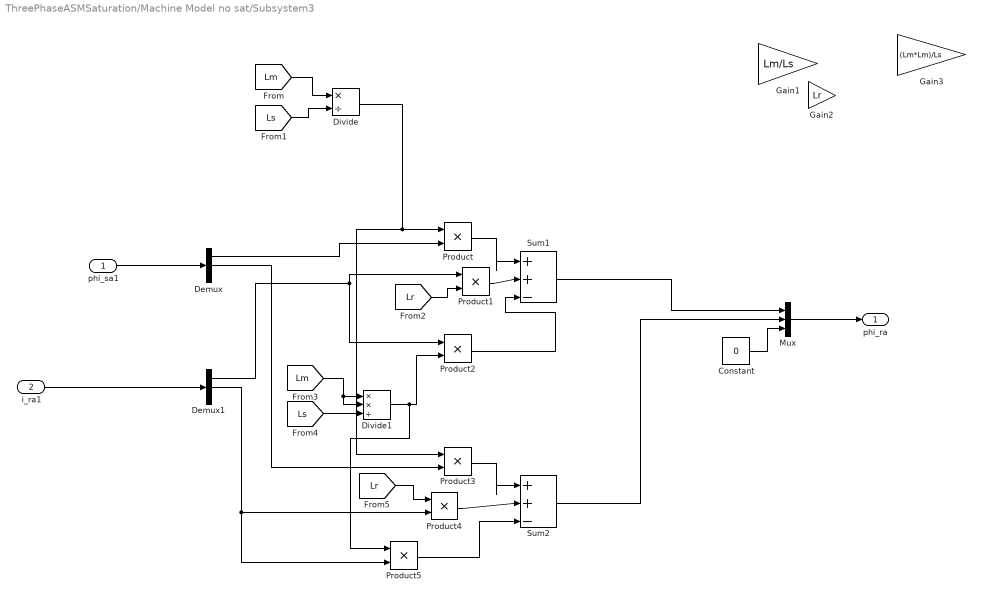
== system ThreePhaseASMSaturation/Machine Model no sat/Subsystem3 ==
  phi_sa1 : Inport
  i_ra1 : Inport  Port=2
  Constant : Constant  Value=0
  Demux : Demux  Outputs=3
  Demux1 : Demux  Outputs=3
  Divide : Product  Inputs=*/
  Divide1 : Product  Inputs=**/
  Gain1 : Gain  Gain=Lm/Ls
  Gain2 : Gain  Gain=Lr
  Gain3 : Gain  Gain=(Lm*Lm)/Ls
  Mux : Mux  Inputs=3
  Product{,1..5} (6 alike) : Product
  Sum1 : Sum  Inputs=|++-  RndMeth=Round
  Sum2 : Sum  Inputs=|++-  RndMeth=Round
  phi_ra : Outport
  wires:
  Product/1 -> Sum1/1
  Product2/1 -> Sum1/3
  Product1/1 -> Sum1/2
  Product3/1 -> Sum2/1
  Product5/1 -> Sum2/3
  Constant/1 -> Mux/3
  phi_sa1/1 -> Demux/1
  i_ra1/1 -> Demux1/1
  Mux/1 -> phi_ra/1
  Demux/1 -> Product/2
  Demux/2 -> Product3/2
  Demux1/1 -> Product2/1, Product1/1
  [Ls] -> Divide/2
  [Lm] -> Divide/1
  Divide/1 -> Product/1, Product3/1
  [Lr] -> Product1/2
  [Ls] -> Divide1/3
  [Lm] -> Divide1/2, Divide1/1
  Divide1/1 -> Product5/1, Product2/2
  Demux1/2 -> Product4/2, Product5/2
  Product4/1 -> Sum2/2
  [Lr] -> Product4/1
  Sum1/1 -> Mux/1
  Sum2/1 -> Mux/2

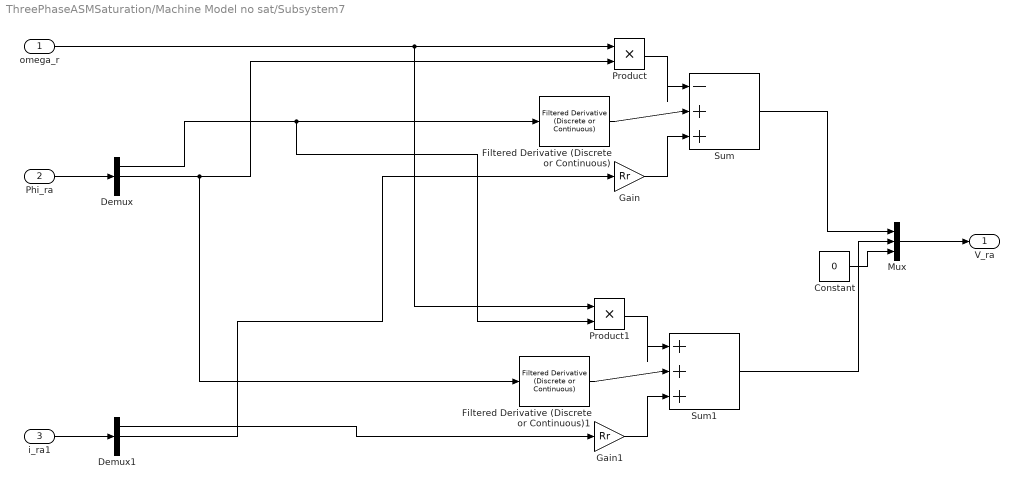
== system ThreePhaseASMSaturation/Machine Model no sat/Subsystem7 ==
  omega_r : Inport
  Phi_ra : Inport  Port=2
  i_ra1 : Inport  Port=3
  Constant : Constant  Value=0
  Demux : Demux  Outputs=3
  Demux1 : Demux  Outputs=3
  Filtered Derivative (Discrete or Continuous) : eeGeneralControl/Filtered Derivative (Discrete or Continuous)  K=1  T=0.1  B=inf  A=-inf  minRatio=10  init_option=Inherited from block input  x0=0  Ts=-1
      settings: LibrarySourceBlock=|
      | ee_sl_lib/General Control/Filtered Derivative
      | (Discrete or Continuous)
  Filtered Derivative (Discrete or Continuous)1 : eeGeneralControl/Filtered Derivative (Discrete or Continuous)  K=1  T=0.1  B=inf  A=-inf  minRatio=10  init_option=Inherited from block input  x0=0  Ts=-1
      settings: LibrarySourceBlock=|
      | ee_sl_lib/General Control/Filtered Derivative
      | (Discrete or Continuous)
  Gain : Gain  Gain=Rr
  Gain1 : Gain  Gain=Rr
  Mux : Mux  Inputs=3
  Product : Product
  Product1 : Product
  Sum : Sum  Inputs=|-++
  Sum1 : Sum  Inputs=|+++
  V_ra : Outport
  wires:
  Product/1 -> Sum/1
  Gain/1 -> Sum/3
  Filtered Derivative (Discrete or Continuous)/1 -> Sum/2
  Gain1/1 -> Sum1/3
  Filtered Derivative (Discrete or Continuous)1/1 -> Sum1/2
  Product1/1 -> Sum1/1
  i_ra1/1 -> Demux1/1
  omega_r/1 -> Product1/1, Product/1
  Demux1/1 -> Gain1/1
  Demux1/2 -> Gain/1
  Phi_ra/1 -> Demux/1
  Demux/2 -> Filtered Derivative (Discrete or Continuous)1/1, Product/2
  Demux/1 -> Product1/2, Filtered Derivative (Discrete or Continuous)/1
  Constant/1 -> Mux/3
  Sum1/1 -> Mux/2
  Sum/1 -> Mux/1
  Mux/1 -> V_ra/1

== system ThreePhaseASMSaturation/Machine Model with sat/D//Q -> d//q1 ==
  i Dr/Qr : Inport
  theta_r (θr) : Inport  Port=2
  Fcn : Fcn  Expr=u[1]*cos(u[3])+u[2]*sin(u[3])
  Fcn1 : Fcn  Expr=-u[1]*sin(u[3])+u[2]*cos(u[3])
  Mux : Mux  Inputs=2
  Mux1 : Mux  Inputs=2
  i dr/qr : Outport  VectorParamsAs1DForOutWhenUnconnected=off
  wires:
  Mux/1 -> i dr/qr/1
  Fcn/1 -> Mux/1
  Fcn1/1 -> Mux/2
  i Dr/Qr/1 -> Mux1/1
  Mux1/1 -> Fcn1/1, Fcn/1
  theta_r (θr)/1 -> Mux1/2

== system ThreePhaseASMSaturation/Machine Model with sat/Just some variable naming stuff ==
  L_m : Inport
  Constant14 : Constant  Value=Lsi
  Constant19 : Constant  Value=Lri
  Constant20 : Constant
  Divide : Product  Inputs=**/
  Product : Product
  Sum : Sum  Inputs=|++
  Sum1 : Sum  Inputs=|++
  Sum2 : Sum  Inputs=|+-
  tag scope: Lr_sat=global, Ls_sat=global, sigma_sat=global
  wires:
  L_m/1 -> Divide/2, Divide/1, Sum/2, Sum1/1
  Constant20/1 -> Sum2/1
  Constant14/1 -> Sum1/2
  Sum/1 -> Product/1, [Lr_sat]
  Divide/1 -> Sum2/2
  Sum2/1 -> [sigma_sat]
  Constant19/1 -> Sum/1
  Sum1/1 -> Product/2, [Ls_sat]
  Product/1 -> Divide/3

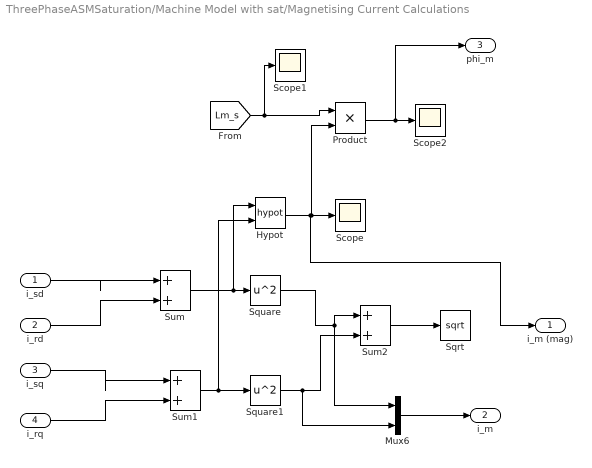
== system ThreePhaseASMSaturation/Machine Model with sat/Magnetising Current Calculations ==
  i_sd : Inport
  i_rd : Inport  Port=2
  i_sq : Inport  Port=3
  i_rq : Inport  Port=4
  Hypot : Math  Operator=hypot
  Mux6 : Mux  Inputs=2
  Product : Product
  Scope : Scope
  Scope1 : Scope
  Scope2 : Scope
  Sqrt : Sqrt
  Square : Math  Operator=square
  Square1 : Math  Operator=square
  Sum : Sum  Inputs=|++
  Sum1 : Sum  Inputs=|++
  Sum2 : Sum  Inputs=|++
  i_m (mag) : Outport
  i_m : Outport  Port=2
  phi_m : Outport  Port=3
  wires:
  Sum/1 -> Hypot/1, Square/1
  Square1/1 -> Mux6/2, Sum2/2
  Sum2/1 -> Sqrt/1
  i_sq/1 -> Sum1/1
  i_rd/1 -> Sum/2
  Square/1 -> Mux6/1, Sum2/1
  Sum1/1 -> Hypot/2, Square1/1
  i_sd/1 -> Sum/1
  Mux6/1 -> i_m/1
  i_rq/1 -> Sum1/2
  Hypot/1 -> i_m (mag)/1, Product/2, Scope/1
  [Lm_s] -> Scope1/1, Product/1
  Product/1 -> phi_m/1, Scope2/1

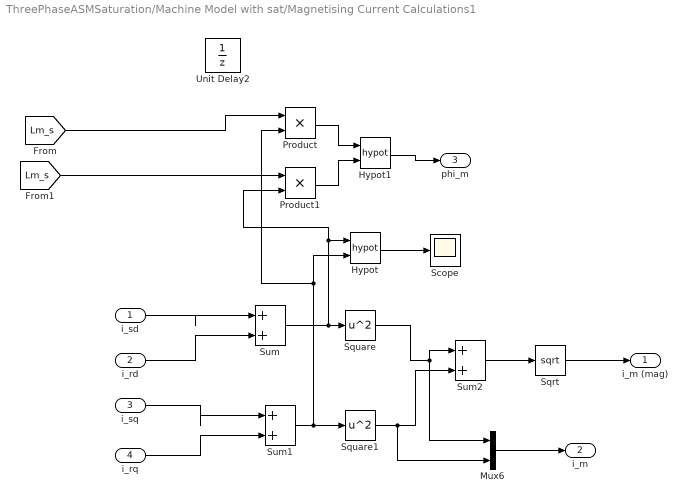
== system ThreePhaseASMSaturation/Machine Model with sat/Magnetising Current Calculations1 ==
  i_sd : Inport
  i_rd : Inport  Port=2
  i_sq : Inport  Port=3
  i_rq : Inport  Port=4
  Hypot : Math  Operator=hypot
  Hypot1 : Math  Operator=hypot
  Mux6 : Mux  Inputs=2
  Product : Product
  Product1 : Product
  Scope : Scope
  Sqrt : Sqrt
  Square : Math  Operator=square
  Square1 : Math  Operator=square
  Sum : Sum  Inputs=|++
  Sum1 : Sum  Inputs=|++
  Sum2 : Sum  Inputs=|++
  Unit Delay2 : UnitDelay  InitialCondition=0.0349  SampleTime=-1  HasFrameUpgradeWarning=on
  i_m (mag) : Outport
  i_m : Outport  Port=2
  phi_m : Outport  Port=3
  wires:
  Sum/1 -> Product1/2, Hypot/1, Square/1
  Square1/1 -> Mux6/2, Sum2/2
  Sum2/1 -> Sqrt/1
  i_sq/1 -> Sum1/1
  i_rd/1 -> Sum/2
  Square/1 -> Mux6/1, Sum2/1
  Sum1/1 -> Product/2, Hypot/2, Square1/1
  i_sd/1 -> Sum/1
  Mux6/1 -> i_m/1
  Sqrt/1 -> i_m (mag)/1
  i_rq/1 -> Sum1/2
  Hypot/1 -> Scope/1
  Product/1 -> Hypot1/1
  Product1/1 -> Hypot1/2
  Hypot1/1 -> phi_m/1
  [Lm_s] -> Product/1
  [Lm_s] -> Product1/1

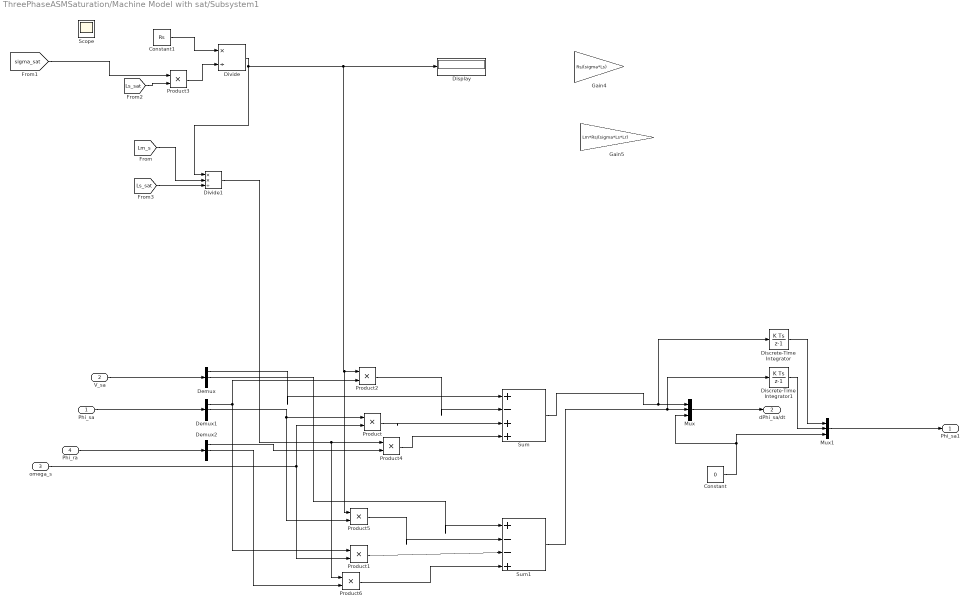
== system ThreePhaseASMSaturation/Machine Model with sat/Subsystem1 ==
  Phi_sa : Inport
  V_sa : Inport  Port=2
  omega_s : Inport  Port=3
  Phi_ra : Inport  Port=4
  Constant : Constant  Value=0
  Constant1 : Constant  Value=Rs
  Demux : Demux  Outputs=3
  Demux1 : Demux  Outputs=3
  Demux2 : Demux  Outputs=3
  Discrete-Time Integrator : DiscreteIntegrator  SampleTime=-1  ICPrevOutput=DiscIntNeverNeededParam  ICPrevScaledInput=DiscIntNeverNeededParam
  Discrete-Time Integrator1 : DiscreteIntegrator  SampleTime=-1  ICPrevOutput=DiscIntNeverNeededParam  ICPrevScaledInput=DiscIntNeverNeededParam
  Display : Display
  Divide : Product  Inputs=*/  OutDataTypeStr=double
  Divide1 : Product  Inputs=**/  OutDataTypeStr=double
  Gain4 : Gain  Gain=Rs/(sigma*Ls)
  Gain5 : Gain  Gain=Lm*Rs/(sigma*Ls*Lr)
  Mux : Mux  Inputs=3
  Mux1 : Mux  Inputs=3
  Product{,1..6} (7 alike) : Product
  Scope : Scope
  Sum : Sum  Inputs=|+-++
  Sum1 : Sum  Inputs=|+--+
  Phi_sa1 : Outport
  dPhi_sa/dt : Outport  Port=2
  wires:
  Product2/1 -> Sum/2
  Product4/1 -> Sum/4
  Product/1 -> Sum/3
  Mux/1 -> dPhi_sa/dt/1
  Demux/1 -> Sum/1
  Product5/1 -> Sum1/2
  Product6/1 -> Sum1/4
  Product1/1 -> Sum1/3
  Demux/2 -> Sum1/1
  Mux1/1 -> Phi_sa1/1
  Demux1/1 -> Product2/2, Product1/1
  Demux2/1 -> Product4/2
  Demux1/2 -> Product5/2, Product/1
  Demux2/2 -> Product6/2
  Constant/1 -> Mux1/3, Mux/3
  Phi_sa/1 -> Demux1/1
  Phi_ra/1 -> Demux2/1
  omega_s/1 -> Product/2, Product1/2
  Sum/1 -> Discrete-Time Integrator/1, Mux/1
  Sum1/1 -> Discrete-Time Integrator1/1, Mux/2
  V_sa/1 -> Demux/1
  [sigma_sat] -> Product3/1
  [Lm_s] -> Divide1/2
  Divide/1 -> Display/1, Product5/1, Product2/1, Divide1/1
  Constant1/1 -> Divide/1
  [Ls_sat] -> Product3/2
  Product3/1 -> Divide/2
  [Ls_sat] -> Divide1/3
  Divide1/1 -> Product6/1, Product4/1
  Discrete-Time Integrator/1 -> Mux1/1
  Discrete-Time Integrator1/1 -> Mux1/2

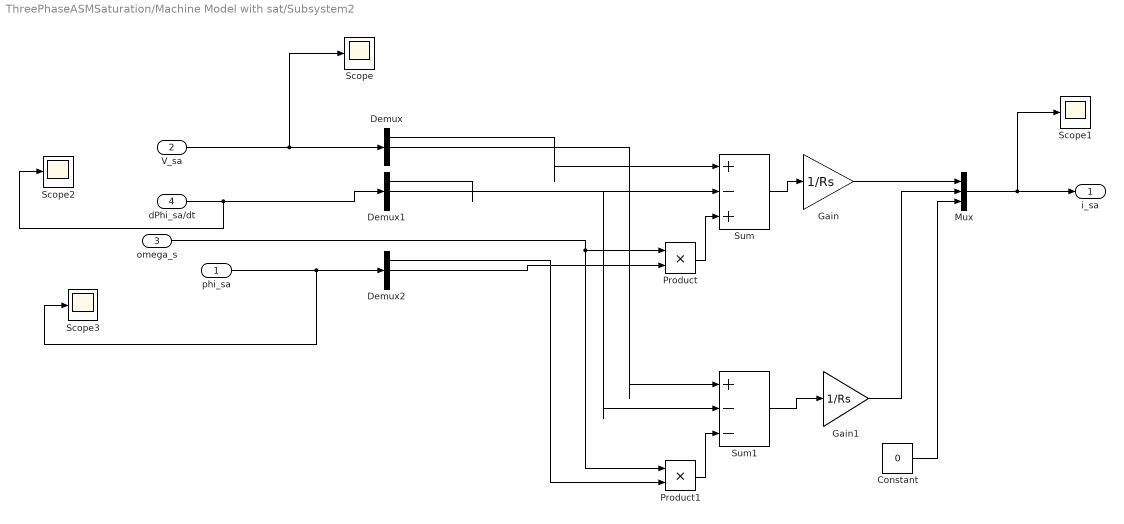
== system ThreePhaseASMSaturation/Machine Model with sat/Subsystem2 ==
  phi_sa : Inport
  V_sa : Inport  Port=2
  omega_s : Inport  Port=3
  dPhi_sa/dt : Inport  Port=4
  Constant : Constant  Value=0
  Demux : Demux  Outputs=3
  Demux1 : Demux  Outputs=3
  Demux2 : Demux  Outputs=3
  Gain : Gain  Gain=1/Rs
  Gain1 : Gain  Gain=1/Rs
  Mux : Mux  Inputs=3
  Product : Product
  Product1 : Product
  Scope{,1..3} (4 alike) : Scope
  Sum : Sum  Inputs=|+-+
  Sum1 : Sum  Inputs=|+--
  i_sa : Outport
  wires:
  Product/1 -> Sum/3
  Constant/1 -> Mux/3
  Demux/1 -> Sum/1
  Demux1/1 -> Sum/2
  Demux2/2 -> Product/2
  Product1/1 -> Sum1/3
  Sum/1 -> Gain/1
  Sum1/1 -> Gain1/1
  Demux/2 -> Sum1/1
  Demux1/2 -> Sum1/2
  Demux2/1 -> Product1/2
  Gain/1 -> Mux/1
  Gain1/1 -> Mux/2
  Mux/1 -> Scope1/1, i_sa/1
  dPhi_sa/dt/1 -> Scope2/1, Demux1/1
  phi_sa/1 -> Scope3/1, Demux2/1
  omega_s/1 -> Product1/1, Product/1
  V_sa/1 -> Scope/1, Demux/1

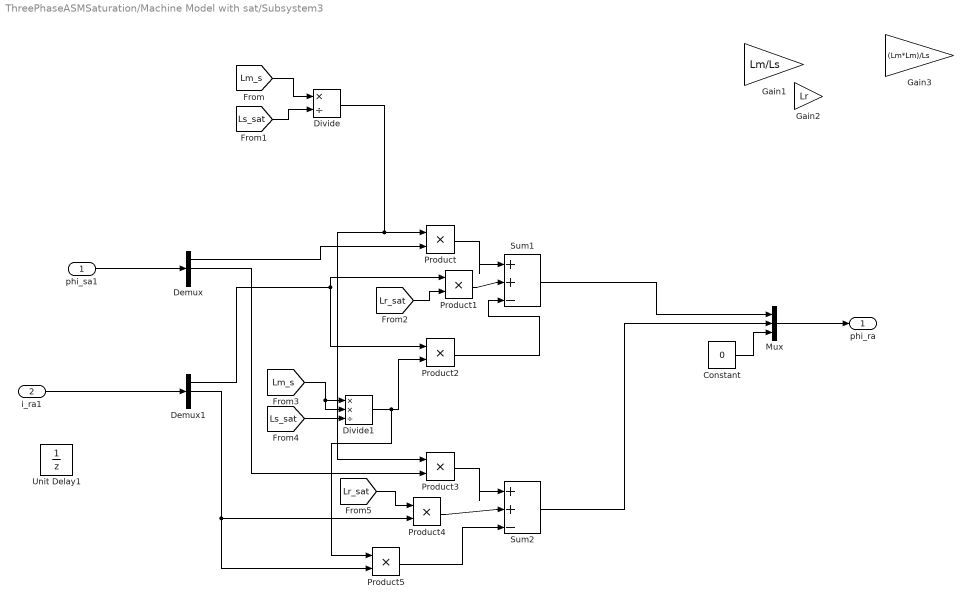
== system ThreePhaseASMSaturation/Machine Model with sat/Subsystem3 ==
  phi_sa1 : Inport
  i_ra1 : Inport  Port=2
  Constant : Constant  Value=0
  Demux : Demux  Outputs=3
  Demux1 : Demux  Outputs=3
  Divide : Product  Inputs=*/
  Divide1 : Product  Inputs=**/
  Gain1 : Gain  Gain=Lm/Ls
  Gain2 : Gain  Gain=Lr
  Gain3 : Gain  Gain=(Lm*Lm)/Ls
  Mux : Mux  Inputs=3
  Product{,1..5} (6 alike) : Product
  Sum1 : Sum  Inputs=|++-  RndMeth=Round
  Sum2 : Sum  Inputs=|++-  RndMeth=Round
  Unit Delay1 : UnitDelay  SampleTime=-1  HasFrameUpgradeWarning=on
  phi_ra : Outport
  wires:
  Product/1 -> Sum1/1
  Product2/1 -> Sum1/3
  Product1/1 -> Sum1/2
  Product3/1 -> Sum2/1
  Product5/1 -> Sum2/3
  Constant/1 -> Mux/3
  phi_sa1/1 -> Demux/1
  Mux/1 -> phi_ra/1
  Demux/1 -> Product/2
  Demux/2 -> Product3/2
  Demux1/1 -> Product2/1, Product1/1
  [Ls_sat] -> Divide/2
  [Lm_s] -> Divide/1
  Divide/1 -> Product/1, Product3/1
  [Lr_sat] -> Product1/2
  [Ls_sat] -> Divide1/3
  [Lm_s] -> Divide1/2, Divide1/1
  Divide1/1 -> Product5/1, Product2/2
  Demux1/2 -> Product4/2, Product5/2
  Product4/1 -> Sum2/2
  [Lr_sat] -> Product4/1
  Sum1/1 -> Mux/1
  Sum2/1 -> Mux/2
  i_ra1/1 -> Demux1/1

== system ThreePhaseASMSaturation/Machine Model with sat/Subsystem7 ==
  omega_r : Inport
  Phi_ra : Inport  Port=2
  i_ra1 : Inport  Port=3
  Constant : Constant  Value=0
  Demux : Demux  Outputs=3
  Demux1 : Demux  Outputs=3
  Filtered Derivative (Discrete or Continuous) : eeGeneralControl/Filtered Derivative (Discrete or Continuous)  K=1  T=0.1  B=inf  A=-inf  minRatio=10  init_option=Inherited from block input  x0=0  Ts=-1
      settings: LibrarySourceBlock=|
      | ee_sl_lib/General Control/Filtered Derivative
      | (Discrete or Continuous)
  Filtered Derivative (Discrete or Continuous)1 : eeGeneralControl/Filtered Derivative (Discrete or Continuous)  K=1  T=0.1  B=inf  A=-inf  minRatio=10  init_option=Inherited from block input  x0=0  Ts=-1
      settings: LibrarySourceBlock=|
      | ee_sl_lib/General Control/Filtered Derivative
      | (Discrete or Continuous)
  Gain : Gain  Gain=Rr
  Gain1 : Gain  Gain=Rr
  Mux : Mux  Inputs=3
  Product : Product
  Product1 : Product
  Sum : Sum  Inputs=|-++
  Sum1 : Sum  Inputs=|+++
  V_ra : Outport
  wires:
  Product/1 -> Sum/1
  Gain/1 -> Sum/3
  Filtered Derivative (Discrete or Continuous)/1 -> Sum/2
  Gain1/1 -> Sum1/3
  Filtered Derivative (Discrete or Continuous)1/1 -> Sum1/2
  Product1/1 -> Sum1/1
  i_ra1/1 -> Demux1/1
  omega_r/1 -> Product1/1, Product/1
  Demux1/1 -> Gain1/1
  Demux1/2 -> Gain/1
  Phi_ra/1 -> Demux/1
  Demux/2 -> Filtered Derivative (Discrete or Continuous)1/1, Product/2
  Demux/1 -> Product1/2, Filtered Derivative (Discrete or Continuous)/1
  Constant/1 -> Mux/3
  Sum1/1 -> Mux/2
  Sum/1 -> Mux/1
  Mux/1 -> V_ra/1
